simulink model "RunwithMOSFET"  (Simulink 7.3)
settings: Solver=ode23t  StartTime=0.0  StopTime=3  RelTol=1e-3
libraries: powerlib x18, simulink x1
settings Model: Creator=lenovo  LastModifiedBy=lenovo

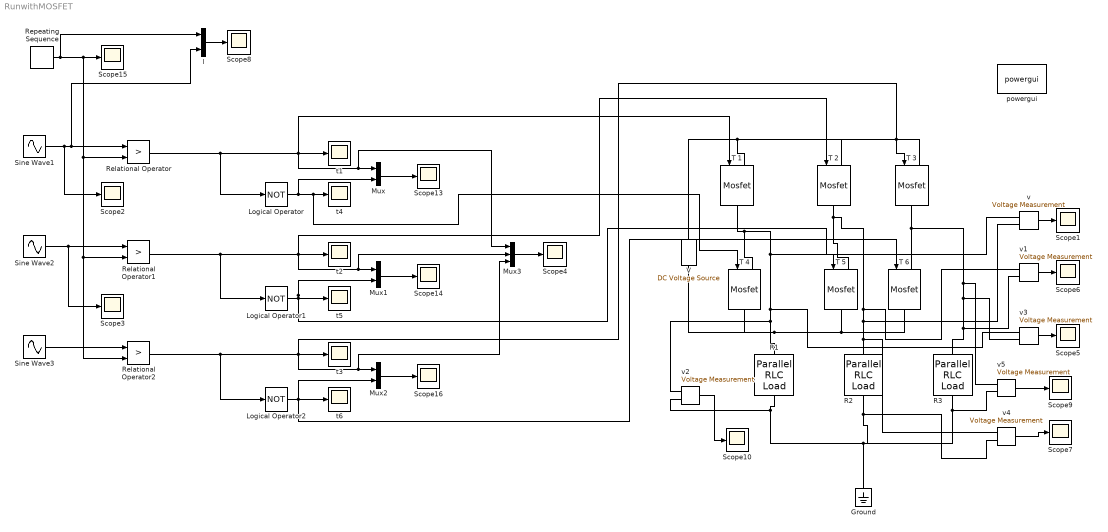
== system RunwithMOSFET ==
  "     R2" : powerlib/Elements/Parallel RLC Load  DialogController=POWERSYS.PowerSysDialog  PhysicalDomain=powersysdomain  SubClassName=unknown  LeftPortType=p1  RightPortType=p1  LConnTagsString=a  RConnTagsString=__new0  NominalVoltage=1000  NominalFrequency=50  ActivePower=10e3  InductivePower=0  CapacitivePower=0  Setx0=off  InitialVoltage=0  SetiL0=off  InitialCurrent=0  Measurements=None
      settings: AttributesFormatString=\n
  Ground : powerlib/Elements/Ground  DialogController=POWERSYS.PowerSysDialog  PhysicalDomain=powersysdomain  SubClassName=unknown  LeftPortType=p1  RightPortType=p1  LConnTagsString=a
  Logical Operator : Logic  Operator=NOT  AllPortsSameDT=off  OutDataTypeMode=boolean  LogicDataType=fixdt(0, 8)  OutDataTypeStr=boolean
  Logical Operator1 : Logic  Operator=NOT  AllPortsSameDT=off  OutDataTypeMode=boolean  LogicDataType=fixdt(0, 8)  OutDataTypeStr=boolean
  Logical Operator2 : Logic  Operator=NOT  AllPortsSameDT=off  OutDataTypeMode=boolean  LogicDataType=fixdt(0, 8)  OutDataTypeStr=boolean
  Mux : Mux  Inputs=2
  Mux1 : Mux  Inputs=2
  Mux2 : Mux  Inputs=2
  Mux3 : Mux  Inputs=3
  R1 : powerlib/Elements/Parallel RLC Load  DialogController=POWERSYS.PowerSysDialog  PhysicalDomain=powersysdomain  SubClassName=unknown  LeftPortType=p1  RightPortType=p1  LConnTagsString=a  RConnTagsString=__new0  NominalVoltage=1000  NominalFrequency=50  ActivePower=10e3  InductivePower=0  CapacitivePower=0  Setx0=off  InitialVoltage=0  SetiL0=off  InitialCurrent=0  Measurements=Branch voltage
      settings: AttributesFormatString=\n
  R3 : powerlib/Elements/Parallel RLC Load  DialogController=POWERSYS.PowerSysDialog  PhysicalDomain=powersysdomain  SubClassName=unknown  LeftPortType=p1  RightPortType=p1  LConnTagsString=a  RConnTagsString=__new0  NominalVoltage=1000  NominalFrequency=50  ActivePower=10e3  InductivePower=0  CapacitivePower=0  Setx0=off  InitialVoltage=0  SetiL0=off  InitialCurrent=0  Measurements=None
      settings: AttributesFormatString=\n
  Relational Operator : RelationalOperator  Operator=>  LogicOutDataTypeMode=boolean  LogicDataType=fixdt(0, 8)  OutDataTypeStr=boolean
  Relational Operator1 : RelationalOperator  Operator=>  LogicOutDataTypeMode=boolean  LogicDataType=fixdt(0, 8)  OutDataTypeStr=boolean
  Relational Operator2 : RelationalOperator  Operator=>  LogicOutDataTypeMode=boolean  LogicDataType=fixdt(0, 8)  OutDataTypeStr=boolean
  Repeating Sequence : simulink/Sources/Repeating Sequence  SystemSampleTime=-1  rep_seq_t=[0 0.1 0.2 0.3 0.4 0.5 0.6 0.7 0.8 0.9 1 1.1 1.2 1.3 1.4 1.5 1.6 1.7 1.8]  rep_seq_y=[1 -1 1 -1 1 -1 1 -1 1 -1 1 -1 1 -1 1 -1 1 -1 1]
  Scope{1..10,13..16} (14 alike) : Scope
      Scope1 settings: YMin=-400  YMax=400  SaveName=ScopeData9
      Scope10 settings: YMin=-400  YMax=400  SaveName=ScopeData19
      Scope13 settings: SaveName=ScopeData6
      Scope14 settings: SaveName=ScopeData7
      Scope16 settings: SaveName=ScopeData8
      Scope2 settings: SaveName=ScopeData13
      Scope3 settings: SaveName=ScopeData14
      Scope4 settings: SaveName=ScopeData15
      Scope5 settings: YMin=-400  YMax=400  SaveName=ScopeData10
      Scope6 settings: YMin=-400  YMax=400  SaveName=ScopeData11
      Scope7 settings: YMin=-400  YMax=400  SaveName=ScopeData16
      Scope8 settings: SaveName=ScopeData17
      Scope9 settings: YMin=-400  YMax=400  SaveName=ScopeData18
  Sine Wave1 : Sin  Amplitude=.5  Bias=0  Frequency=3.3333333  Phase=0  Samples=10  SampleTime=0  Offset=0
  Sine Wave2 : Sin  Amplitude=.5  Bias=0  Frequency=3.3333333  Phase=-2.09  Samples=10  SampleTime=0  Offset=0
  Sine Wave3 : Sin  Amplitude=.5  Bias=0  Frequency=5.3333333  Phase=-4.18  Samples=10  SampleTime=0  Offset=0
  T {1..6} (6 alike) : powerlib/Power Electronics/Mosfet  DialogController=POWERSYS.PowerSysDialog  SystemSampleTime=-1  Ron=0.1  Lon=0  Rd=0.01  Vfd=0  IC=0  Rs=1e5  Cs=inf  Measurements=off
  V : powerlib/Electrical Sources/DC Voltage Source  DialogController=POWERSYS.PowerSysDialog  SystemSampleTime=-1  Amplitude=300  Measurements=Voltage
  l : Concatenate  Mode=Vector
  powergui : powerlib/powergui  Priority=1  SystemSampleTime=-1  SimulationMode=Continuous  SampleTime=50e-6  frequency=60  SPID=off  DisableSnubberDevices=off  DisableRonSwitches=off  DisableVfSwitches=off  SwTol=0  Interpol=off  frequencyindice=0  echomessages=off  HookPort=off  DisplayEquations=off  FunctionMessages=off  EnableUseOfTLC=off  x0status=blocks  RestoreLinks=warning  Frange=[0:2:500]  Ylog=off  Xlog=on  ShowGrid=off  save=off  variable=ZData  ZoomFFT=on  StartTime=0.0  cycles=1  DisplayStyle=1  fundamental=60  FreqAxis=off  MaxFrequency=1000  frequencyindicesteady=1  RmsSteady=1  display=off  Ts=0  methode=off
  t{1..6} (6 alike) : Scope
      t1 settings: SaveName=ScopeData12
      t3 settings: SaveName=ScopeData2
      t4 settings: SaveName=ScopeData3
      t5 settings: SaveName=ScopeData4
      t6 settings: SaveName=ScopeData5
  v{,1..5} (6 alike) : powerlib/Measurements/Voltage Measurement  DialogController=POWERSYS.PowerSysDialog  SystemSampleTime=-1  PhasorSimulation=off  OutputType=Complex  PSBequivalent=0
  wires:
  Sine Wave1/1 -> Scope2/1, Relational Operator/1, l/2
  Sine Wave2/1 -> Relational Operator1/1, Scope3/1
  Sine Wave3/1 -> Relational Operator2/1
  Relational Operator/1 -> Logical Operator/1, t1/1, Mux/1, Mux3/1, T 1/1
  Relational Operator1/1 -> Logical Operator1/1, t2/1, Mux1/1, Mux3/2, T 2/1
  Relational Operator2/1 -> Logical Operator2/1, t3/1, Mux2/1, Mux3/3, T 3/1
  Logical Operator/1 -> Mux/2, t4/1, T 4/1
  Logical Operator1/1 -> t5/1, Mux1/2, T 5/1
  Logical Operator2/1 -> Mux2/2, t6/1, T 6/1
  Mux1/1 -> Scope14/1
  Mux2/1 -> Scope16/1
  Mux/1 -> Scope13/1
  Repeating Sequence/1 -> Relational Operator/2, Relational Operator2/2, Relational Operator1/2, Scope15/1, l/1
  Mux3/1 -> Scope4/1
  v/1 -> Scope1/1
  v1/1 -> Scope6/1
  v3/1 -> Scope5/1
  v2/1 -> Scope10/1
  v4/1 -> Scope7/1
  v5/1 -> Scope9/1
  l/1 -> Scope8/1
  connections:
  T 3/LConn1 -- V/RConn1 -- T 1/LConn1 -- T 2/LConn1
  v4/LConn2 -- "     R2"/RConn1 -- Ground/LConn1 -- R1/RConn1 -- v2/LConn2 -- R3/RConn1 -- v5/LConn2
  v5/LConn1 -- T 3/RConn1 -- T 6/LConn1 -- v3/LConn2 -- v1/LConn2 -- R3/LConn1
  v4/LConn1 -- "     R2"/LConn1 -- v1/LConn1 -- T 2/RConn1 -- T 5/LConn1 -- v/LConn2
  T 6/RConn1 -- V/LConn1 -- T 4/RConn1 -- T 5/RConn1
  R1/LConn1 -- v3/LConn1 -- T 1/RConn1 -- T 4/LConn1 -- v/LConn1 -- v2/LConn1
